simulink model "Pendulum"  (Simulink 8.4)
settings: Solver=ode4  StartTime=0.0  StopTime=9.99  FixedStep=T_s  RelTol=1e-3
PreLoadFcn:
  | Pendulum
undefined symbols (not defined in the file or in its folder): d, g, kfp
settings Model: Creator=mueller  LastModifiedBy=Vincent

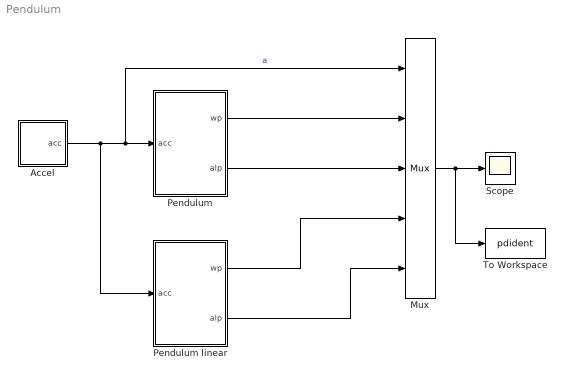
== system Pendulum ==
  Accel : Subsystem
  Mux : Mux  Inputs=5
  Pendulum : Subsystem
  Pendulum linear : Subsystem
  Scope : Scope
      settings: TimeRange=10  YMin=-2  YMax=4
  To Workspace : ToWorkspace  VariableName=pdident  SampleTime=-1
  wires:
  Mux/1 -> Scope/1, To Workspace/1
  Pendulum/2(alp) -> Mux/3
  Pendulum/1(wp) -> Mux/2
  Accel/1(acc) -> Mux/1, Pendulum/1(acc), Pendulum linear/1(acc)  "a"
  Pendulum linear/1(wp) -> Mux/4
  Pendulum linear/2(alp) -> Mux/5

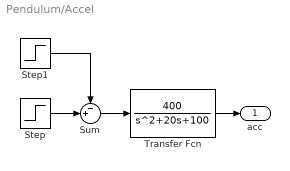
== system Pendulum/Accel ==
  Step : Step  Time=0.1  SampleTime=0
  Step1 : Step  SampleTime=0
  Sum : Sum  Inputs=-+|
  Transfer Fcn : TransferFcn  Numerator=400  Denominator=[1 20 100]
  acc : Outport
  wires:
  Step1/1 -> Sum/1
  Step/1 -> Sum/2
  Sum/1 -> Transfer Fcn/1
  Transfer Fcn/1 -> acc/1

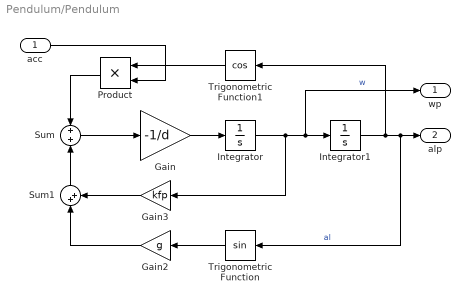
== system Pendulum/Pendulum ==
  acc : Inport
  Gain : Gain  Gain=-1/d
  Gain2 : Gain  Gain=g
  Gain3 : Gain  Gain=kfp
  Integrator : Integrator
  Integrator1 : Integrator
  Product : Product  RndMeth=Zero
  Sum : Sum  Inputs=+|+
  Sum1 : Sum  Inputs=|++
  Trigonometric Function : Trigonometry
  Trigonometric Function1 : Trigonometry  Operator=cos
  wp : Outport
  alp : Outport  Port=2
  wires:
  Integrator/1 -> Integrator1/1, wp/1, Gain3/1  "w"
  Gain/1 -> Integrator/1
  Integrator1/1 -> Trigonometric Function1/1, Trigonometric Function/1, alp/1  "al"
  Trigonometric Function1/1 -> Product/1
  Trigonometric Function/1 -> Gain2/1
  Product/1 -> Sum/1
  Sum/1 -> Gain/1
  Sum1/1 -> Sum/2
  Gain3/1 -> Sum1/2
  Gain2/1 -> Sum1/1
  acc/1 -> Product/2

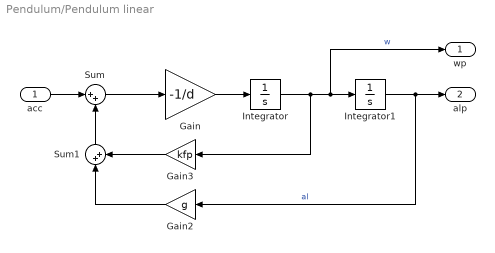
== system Pendulum/Pendulum linear ==
  acc : Inport
  Gain : Gain  Gain=-1/d
  Gain2 : Gain  Gain=g
  Gain3 : Gain  Gain=kfp
  Integrator : Integrator
  Integrator1 : Integrator
  Sum : Sum  Inputs=|++
  Sum1 : Sum  Inputs=|++
  wp : Outport
  alp : Outport  Port=2
  wires:
  Integrator/1 -> Integrator1/1, wp/1, Gain3/1  "w"
  Gain/1 -> Integrator/1
  Sum/1 -> Gain/1
  Sum1/1 -> Sum/2
  Gain3/1 -> Sum1/2
  Gain2/1 -> Sum1/1
  Integrator1/1 -> alp/1, Gain2/1  "al"
  acc/1 -> Sum/1
